simulink model "CP3_1"  (R2020a)
settings: Solver=VariableStepAuto  StartTime=0.0  StopTime=3  RelTol=1e-3
model workspace (MAT data in the model file):
  L = 1
  gamma = 1
  kh = 1
  kv = 1
  v = 1
  xg = 1
settings Model: Creator=fould  LastModifiedBy=fould

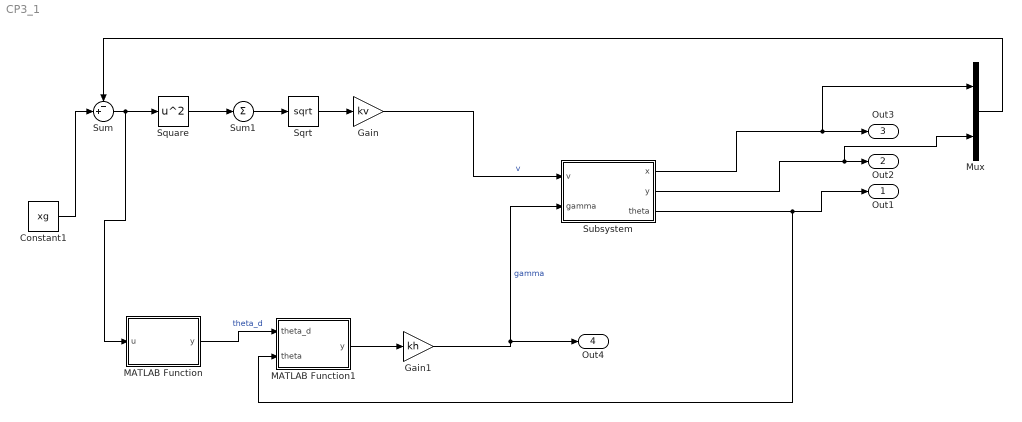
== system CP3_1 ==
  Constant1 : Constant  Value=xg
  Gain : Gain  Gain=kv
  Gain1 : Gain  Gain=kh
  MATLAB Function : MATLAB Function  TreatAsAtomicUnit=on
  MATLAB Function1 : MATLAB Function  TreatAsAtomicUnit=on
  Mux : Mux  Inputs=2
  Sqrt : Sqrt  SaturateOnIntegerOverflow=on
  Square : Math  Operator=square  SaturateOnIntegerOverflow=on
  Subsystem : Subsystem
  Sum : Sum  Inputs=-+|
  Sum1 : Sum  Inputs=|+|
  Out1 : Outport  SignalName=theta
  Out2 : Outport  Port=2  SignalName=y
  Out3 : Outport  Port=3  SignalName=x
  Out4 : Outport  Port=4  SignalName=gamma
  wires:
  Subsystem/1(x) -> Mux/1, Out3/1
  Subsystem/2(y) -> Mux/2, Out2/1
  Subsystem/3(theta) -> MATLAB Function1/2(theta), Out1/1
  Sum/1 -> MATLAB Function/1(u), Square/1
  Square/1 -> Sum1/1
  Sum1/1 -> Sqrt/1
  Sqrt/1 -> Gain/1
  Gain/1 -> Subsystem/1(v)  "v"
  Constant1/1 -> Sum/2
  Mux/1 -> Sum/1
  MATLAB Function/1(y) -> MATLAB Function1/1(theta_d)  "theta_d"
  MATLAB Function1/1(y) -> Gain1/1
  Gain1/1 -> Out4/1, Subsystem/2(gamma)  "gamma"

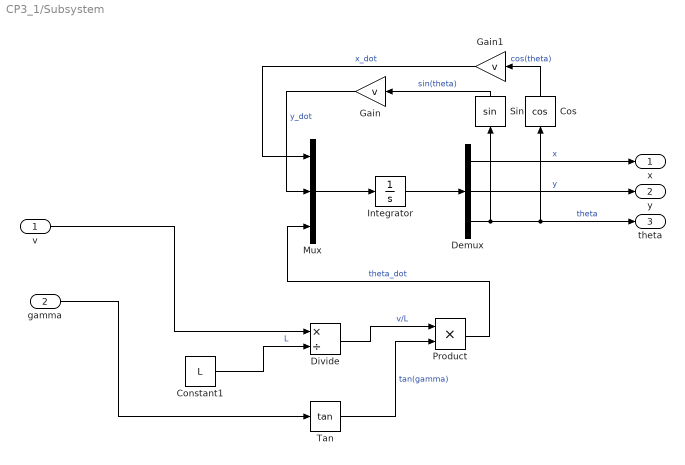
== system CP3_1/Subsystem ==
  v : Inport
  gamma : Inport  Port=2
  Constant1 : Constant  Value=L
  Cos : Trigonometry  Operator=cos
  Demux : Demux  Outputs=3
  Divide : Product  Inputs=*/
  Gain : Gain  Gain=v
  Gain1 : Gain  Gain=v
  Integrator : Integrator
  Mux : Mux  Inputs=3
  Product : Product
  Sin : Trigonometry
  Tan : Trigonometry  Operator=tan
  x : Outport
  y : Outport  Port=2
  theta : Outport  Port=3
  wires:
  Tan/1 -> Product/2  "tan(gamma)"
  Divide/1 -> Product/1  "v/L"
  Demux/3 -> theta/1, Cos/1, Sin/1  "theta"
  Gain1/1 -> Mux/1  "x_dot"
  Integrator/1 -> Demux/1
  Gain/1 -> Mux/2  "y_dot"
  Constant1/1 -> Divide/2  "L"
  gamma/1 -> Tan/1
  Mux/1 -> Integrator/1
  Sin/1 -> Gain/1  "sin(theta)"
  Cos/1 -> Gain1/1  "cos(theta)"
  Product/1 -> Mux/3  "theta_dot"
  v/1 -> Divide/1
  Demux/2 -> y/1  "y"
  Demux/1 -> x/1  "x"

== matlab function CP3_1/MATLAB Function ==
  data: u input; y output
function y = fcn(u)

y = atan2(u(2),u(1));

== matlab function CP3_1/MATLAB Function1 ==
  data: theta_d input; y output; theta input
function y = fcn(theta_d,theta)

y = angdiff(theta_d,theta);
